simulink library "INT_InjCrv_PiI2"  (R2016b)
settings: Solver=VariableStepAuto  StartTime=0.0  StopTime=10.0  RelTol=1e-3
settings Model: Creator=mayongchao  LastModifiedBy=mayongchao

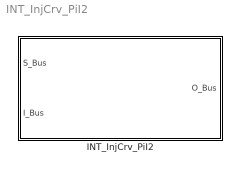
== system INT_InjCrv_PiI2 ==
  INT_InjCrv_PiI2 : Subsystem

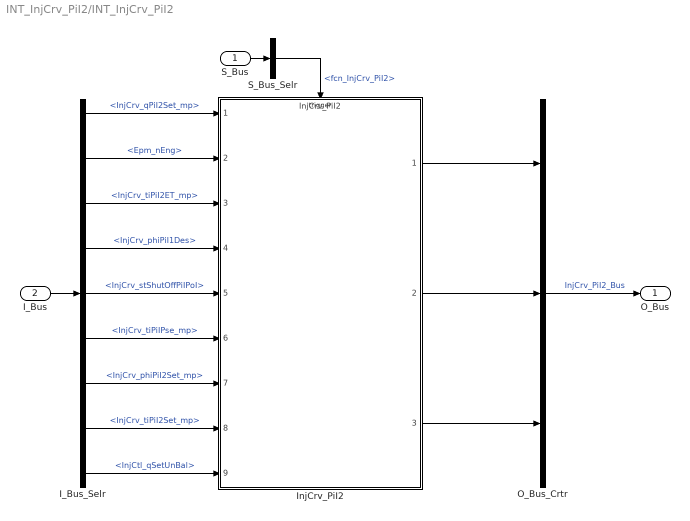
== system INT_InjCrv_PiI2/INT_InjCrv_PiI2 ==
  S_Bus : Inport
  I_Bus : Inport  Port=2
  I_Bus_Selr : BusSelector  OutputSignals=InjCrv_qPiI2Set_mp,Epm_nEng,InjCrv_tiPiI2ET_mp,InjCrv_phiPiI1Des,InjCrv_stShutOffPiIPoI,InjCrv_tiPiIPse_mp,InjCrv_phiPiI2Set_mp,InjCrv_tiPiI2Set_mp,InjCtl_qSetUnBal
  InjCrv_PiI2 : ModelReference  ModelNameDialog=InjCrv_PiI2  SimulationMode=Normal  ModelReferenceVersion=1.36  TriggerPortName=function  TriggerPortTriggerType=function-call  TriggerPortStatesWhenEnabling=held
  O_Bus_Crtr : BusCreator  Inputs=3
  S_Bus_Selr : BusSelector  OutputSignals=fcn_InjCrv_PiI2
  O_Bus : Outport
  wires:
  S_Bus_Selr/1 -> InjCrv_PiI2/Trigger  "<fcn_InjCrv_PiI2>"
  S_Bus/1 -> S_Bus_Selr/1
  I_Bus/1 -> I_Bus_Selr/1
  I_Bus_Selr/1 -> InjCrv_PiI2/1  "<InjCrv_qPiI2Set_mp>"
  I_Bus_Selr/2 -> InjCrv_PiI2/2  "<Epm_nEng>"
  I_Bus_Selr/3 -> InjCrv_PiI2/3  "<InjCrv_tiPiI2ET_mp>"
  I_Bus_Selr/4 -> InjCrv_PiI2/4  "<InjCrv_phiPiI1Des>"
  I_Bus_Selr/5 -> InjCrv_PiI2/5  "<InjCrv_stShutOffPiIPoI>"
  I_Bus_Selr/6 -> InjCrv_PiI2/6  "<InjCrv_tiPiIPse_mp>"
  I_Bus_Selr/7 -> InjCrv_PiI2/7  "<InjCrv_phiPiI2Set_mp>"
  I_Bus_Selr/8 -> InjCrv_PiI2/8  "<InjCrv_tiPiI2Set_mp>"
  I_Bus_Selr/9 -> InjCrv_PiI2/9  "<InjCtl_qSetUnBal>"
  O_Bus_Crtr/1 -> O_Bus/1  "InjCrv_PiI2_Bus"
  InjCrv_PiI2/1 -> O_Bus_Crtr/1
  InjCrv_PiI2/2 -> O_Bus_Crtr/2
  InjCrv_PiI2/3 -> O_Bus_Crtr/3
